simulink model "temp_pid"  (R2018a)
settings: Solver=FixedStepAuto  StartTime=0.0  StopTime=20000  FixedStep=1  RelTol=1e-3
undefined symbols (not defined in the file): daq
libraries: daqlib x2, simulink x1
settings Model: Creator=matthew  LastModifiedBy=matthew

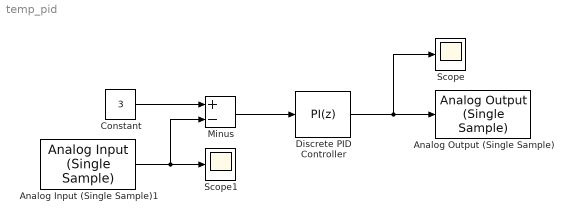
== system temp_pid ==
  Analog Input (Single Sample)1 : daqlib/Analog Input (Single Sample)  DeviceMenu=ni myDAQ1 (NI myDAQ)  Device=ni myDAQ1 (NI myDAQ)  ObjConstructor=daq.createSession('ni')  BlockSampleTime=1  NChannelsSelected=1  Channels=1$ai0$$myDAQ1$1$2$1$1$#0$ai1$$myDAQ1$1$1$1$1$#  NPorts=1 for all channels  OutputTimestamp=off
      settings: SourceProductName=Data Acquisition Toolbox  SourceProductBaseCode=DA
  Analog Output (Single Sample) : daqlib/Analog Output (Single Sample)  DeviceMenu=ni myDAQ1 (NI myDAQ)  Device=ni myDAQ1 (NI myDAQ)  ObjConstructor=daq.createSession('ni')  NChannelsSelected=1  Channels=1$ao0$$myDAQ1$1$2$N/A$#0$ao1$$myDAQ1$1$2$N/A$#  NPorts=1 for all channels  BlockSampleTime=1
      settings: SourceProductName=Data Acquisition Toolbox  SourceProductBaseCode=DA
  Constant : Constant  Value=3
  Discrete PID Controller : simulink/Continuous/PID Controller  Controller=PI  TimeDomain=Discrete-time  SampleTime=-1  IntegratorMethod=Forward Euler  FilterMethod=Forward Euler  Form=Parallel  UseFilter=on  ControllerParametersSource=internal  P=1  I=0.1  D=0  N=10  InitialConditionSource=internal  InitialConditionForIntegrator=0  InitialConditionForFilter=0  ExternalReset=none  LimitOutput=on  UpperSaturationLimit=10  LowerSaturationLimit=0  LinearizeAsGain=off  AntiWindupMode=clamping  Kb=1  TrackingMode=off  Kt=1  PParamMin=[]  PParamMax=[]  IParamMin=[]  IParamMax=[]  DParamMin=[]  DParamMax=[]  NParamMin=[]  NParamMax=[]  KbParamMin=[]  KbParamMax=[]  KtParamMin=[]  KtParamMax=[]  POutMin=[]  POutMax=[]  IOutMin=[]  IOutMax=[]  DOutMin=[]  DOutMax=[]  NOutMin=[]  NOutMax=[]  KbOutMin=[]  KbOutMax=[]  KtOutMin=[]  KtOutMax=[]  IntegratorOutMin=[]  IntegratorOutMax=[]  FilterOutMin=[]  FilterOutMax=[]  SumOutMin=[]  SumOutMax=[]  SumI1OutMin=[]  SumI1OutMax=[]  SumI2OutMin=[]  SumI2OutMax=[]  SumI3OutMin=[]  SumI3OutMax=[]  SumDOutMin=[]  SumDOutMax=[]  SaturationOutMin=[]  SaturationOutMax=[]  IntegratorContinuousStateAttributes=''  IntegratorStateMustResolveToSignalObject=off  IntegratorRTWStateStorageClass=Auto  FilterContinuousStateAttributes=''  FilterStateMustResolveToSignalObject=off  FilterRTWStateStorageClass=Auto  DifferentiatorICPrevScaledInput=0  DifferentiatorOutMin=[]  DifferentiatorOutMax=[]  FilterDiffOutCoefMin=[]  FilterDiffOutCoefMax=[]  SumDenOutMin=[]  SumDenOutMax=[]  SumNumOutMin=[]  SumNumOutMax=[]  ReciprocalOutMin=[]  ReciprocalOutMax=[]  DivideOutMin=[]  DivideOutMax=[]  TunerSelectOption=Transfer Function Based (PID Tuner App)
  Minus : Sum  Inputs=+-
  Scope : Scope
  Scope1 : Scope
  wires:
  Minus/1 -> Discrete PID Controller/1
  Constant/1 -> Minus/1
  Analog Input (Single Sample)1/1 -> Scope1/1, Minus/2
  Discrete PID Controller/1 -> Scope/1, Analog Output (Single Sample)/1
